simulink model "bai11"  (R2022b)
settings: Solver=VariableStepAuto  StartTime=0.0  StopTime=10.0  RelTol=1e-3
settings Model: Creator=admin  LastModifiedBy=admin

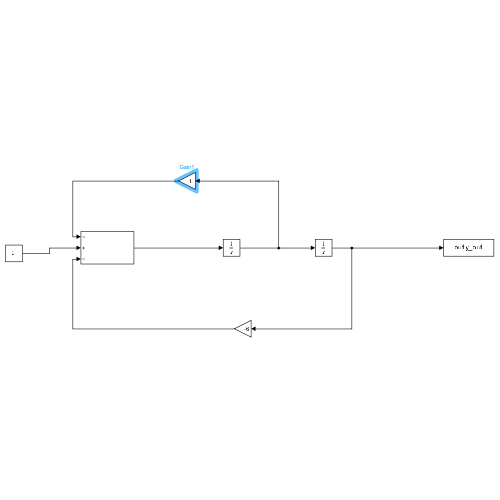
[thumbnail: Simulink's stored preview of the top-level diagram]
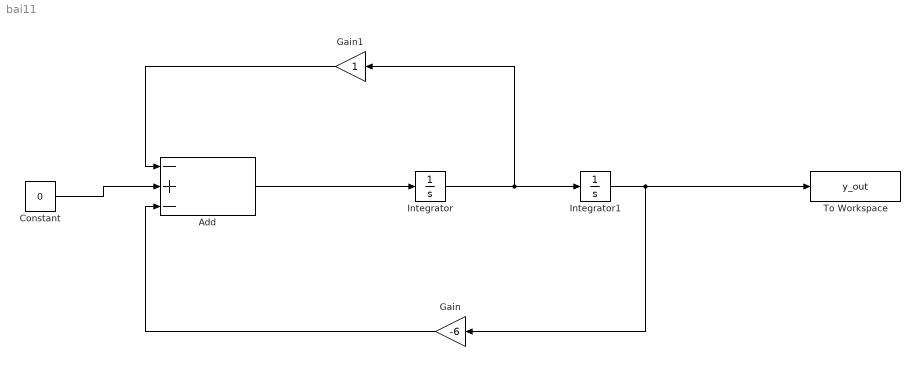
== system bai11 ==
  Add : Sum  Inputs=-+-
  Constant : Constant  Value=0
  Gain : Gain  Gain=-6
  Gain1 : Gain
  Integrator : Integrator  InitialCondition=5
  Integrator1 : Integrator  InitialCondition=4
  To Workspace : ToWorkspace  VariableName=y_out  SaveFormat=Structure With Time  SampleTime=-1
  wires:
  Constant/1 -> Add/2
  Gain1/1 -> Add/1
  Add/1 -> Integrator/1
  Integrator/1 -> Gain1/1, Integrator1/1
  Integrator1/1 -> Gain/1, To Workspace/1
  Gain/1 -> Add/3
